simulink model "mySAD_project_full_mission"  (R2023b)
settings: Solver=ode4  StartTime=0.0  StopTime=tf  FixedStep=t_step  RelTol=1e-3
values from neighbouring files (symbols this model uses):
  A1 = importdata("igrfSg.txt")    [SAD_project_code.m]
  A2 = importdata("igrfSh.txt")    [SAD_project_code.m]
  A_1 = area_face(1)    [SAD_project_code.m]
  A_2 = area_face(2)    [SAD_project_code.m]
  A_3 = area_face(3)    [SAD_project_code.m]
  A_4 = area_face(4)    [SAD_project_code.m]
  A_5 = area_face(5)    [SAD_project_code.m]
  A_6 = area_face(6)    [SAD_project_code.m]
  alpha = [1/6 5/6]    [SAD_project_code.m]
  DCM_eci_per = rotationMatrix(rad2deg(i),rad2deg(OM), rad2deg(om))    [SAD_project_code.m]
  e = 0.0011241    [SAD_project_code.m]
  FS = 50000e-9    (= 5e-05)    [SAD_project_code.m]
  H0 = [g_10 g_11 h_11]'    [SAD_project_code.m]
  h_r_0 = [0,0,0]'    [SAD_project_code.m]
  horizon_cone_limit = deg2rad(350)    [SAD_project_code.m]
  I = 5/12.*diag([Ix Iy Iz])    [SAD_project_code.m]
  i = deg2rad(97.55)    [SAD_project_code.m]
  I_inv = inv(I)    [SAD_project_code.m]
  I_RW = 1e-2    (= 0.01)    [SAD_project_code.m]
  I_vector_RW = [I_RW I_RW I_RW]'    [SAD_project_code.m]
  inc_tot = sqrt(inc_lin^2 + inc_acc^2)    [SAD_project_code.m]
  InitialTrueAnomalyOfEarth = 0    [SAD_project_code.m]
  j_b = [0.001 0.005 0.001]'    [SAD_project_code.m]
  K1_point = lqr(A, B, Q, R)    [SAD_project_code.m]
  K1_slew = lqr(A,B, Q, R)    [SAD_project_code.m]
  K2_point = K1_point.^2/2    [SAD_project_code.m]
  K2_slew = K1_slew.^2/2    [SAD_project_code.m]
  K_detumbling = lqr(A,B,Q,R)    [SAD_project_code.m]
  matrix_RW_config = eye(3)    [SAD_project_code.m]
  matrix_RW_config_inv = inv(matrix_RW_config)    [SAD_project_code.m]
  mu_E = astroConstants(13)    [SAD_project_code.m]
  N_1 = BODY(1,:)    [SAD_project_code.m]
  N_2 = BODY(2,:)    [SAD_project_code.m]
  N_3 = BODY(3,:)    [SAD_project_code.m]
  N_4 = BODY(4,:)    [SAD_project_code.m]
  N_5 = BODY(5,:)    [SAD_project_code.m]
  N_6 = BODY(6,:)    [SAD_project_code.m]
  n_e = sqrt(mu_E/a^3)    [SAD_project_code.m]
  N_order = 4    [SAD_project_code.m]
  om = deg2rad(206.3209)    [SAD_project_code.m]
  OM = deg2rad(50.7464)    [SAD_project_code.m]
  p = a*(1-e^2)    [SAD_project_code.m]
  q0 = [0.1, -0.7, 0.51, 0.41]    [SAD_project_code.m]
  r_1 = r(1,:)    [SAD_project_code.m]
  r_2 = r(2,:)    [SAD_project_code.m]
  r_3 = r(3,:)    [SAD_project_code.m]
  r_4 = r(4,:)    [SAD_project_code.m]
  r_5 = r(5,:)    [SAD_project_code.m]
  r_6 = r(6,:)    [SAD_project_code.m]
  R_E = astroConstants(23)    [SAD_project_code.m]
  rho_d1 = 0.1    [SAD_project_code.m]
  rho_d2 = 0.1    [SAD_project_code.m]
  rho_d3 = 0.1    [SAD_project_code.m]
  rho_d4 = 0.1    [SAD_project_code.m]
  rho_d5 = 0.1    [SAD_project_code.m]
  rho_d6 = 0.1    [SAD_project_code.m]
  rho_s1 = rho_s(1)    [SAD_project_code.m]
  rho_s2 = rho_s(2)    [SAD_project_code.m]
  rho_s3 = rho_s(3)    [SAD_project_code.m]
  rho_s4 = rho_s(4)    [SAD_project_code.m]
  rho_s5 = rho_s(5)    [SAD_project_code.m]
  rho_s6 = rho_s(6)    [SAD_project_code.m]
  t_step = 0.01    [SAD_project_code.m]
  th0 = deg2rad(0)    [SAD_project_code.m]
  timeoflaunch = date2mjd2000(date0)    [SAD_project_code.m]
  torque_max = 0.8    [SAD_project_code.m]
  ts_sensor = 5*t_step    (= 0.05)    [SAD_project_code.m]
  w0 = [wx0 wy0 wz0]'    [SAD_project_code.m]
  w0_RW = [0 0 0]    [SAD_project_code.m]
  w_E = deg2rad(15.04)/60/60    [SAD_project_code.m]
  wMax_RW = 2*pi * RPM_max_RW / 60    (= 527.263967027)    [SAD_project_code.m]
libraries: matrix_library x31, simulink_extras x6, sharedtransform x5, simulink x3, dspindex x3, vrlib x2, dspinverses x1, aerolibutil x1
(part 2 of 4)

== system mySAD_project_full_mission/Reaction Wheel Actuator/detect if the RW is saturated (output == 1 isSaturated) ==
  w : Inport
  Abs : Abs  SaturateOnIntegerOverflow=off
  Compare To Constant : simulink/Logic and Bit Operations/Compare To Constant  relop=>=  const=wMax_RW  OutDataTypeStr=boolean
  Demux : Demux  Outputs=3
  Logical Operator : Logic  Operator=OR  AllPortsSameDT=off  OutDataTypeStr=boolean
  Logical Operator1 : Logic  Operator=OR  AllPortsSameDT=off  OutDataTypeStr=boolean
  Logical Operator2 : Logic  Operator=OR  AllPortsSameDT=off  OutDataTypeStr=boolean
  Unit Delay : UnitDelay  SampleTime=-1  HasFrameUpgradeWarning=on
  Unit Delay2 : UnitDelay  SampleTime=-1  HasFrameUpgradeWarning=on
  Unit Delay4 : UnitDelay  SampleTime=-1  HasFrameUpgradeWarning=on
  flag RW1 : Outport
  flag RW2 : Outport  Port=2
  flag RW3 : Outport  Port=3
  wires:
  Unit Delay4/1 -> Logical Operator2/2
  Unit Delay/1 -> Logical Operator/2
  Demux/1 -> Logical Operator/1
  Logical Operator/1 -> flag RW1/1, Unit Delay/1
  Unit Delay2/1 -> Logical Operator1/2
  Logical Operator2/1 -> flag RW3/1, Unit Delay4/1
  Demux/2 -> Logical Operator1/1
  Logical Operator1/1 -> flag RW2/1, Unit Delay2/1
  Demux/3 -> Logical Operator2/1
  Abs/1 -> Compare To Constant/1
  w/1 -> Abs/1
  Compare To Constant/1 -> Demux/1

== system mySAD_project_full_mission/Attitude determination and sensoring/Horizon Sensor1/Normalize Vector1 ==
  Vector : Inport
  Divide : Product  Inputs=*/
  Normalize Vector : Subsystem  AncestorBlock=LibrarySAD5/Normalize Vector1
  Versor : Outport
  wires:
  Vector/1 -> Normalize Vector/1(Vector), Divide/1
  Divide/1 -> Versor/1
  Normalize Vector/1(Norm) -> Divide/2

== system mySAD_project_full_mission/Attitude determination and sensoring/Horizon Sensor1/Normalize Vector2 ==
  Vector : Inport
  Divide : Product  Inputs=*/
  Normalize Vector : Subsystem  AncestorBlock=LibrarySAD5/Normalize Vector1
  Versor : Outport
  wires:
  Vector/1 -> Normalize Vector/1(Vector), Divide/1
  Divide/1 -> Versor/1
  Normalize Vector/1(Norm) -> Divide/2

== system mySAD_project_full_mission/Attitude determination and sensoring/Horizon Sensor1/True Roll and Pitch betwen nadir and -z_body ==
  note: credo inutili e sbagliati
  R_b : Inport
  cone_limit_angle : Inport  Port=2
  Abs2 : Abs  SaturateOnIntegerOverflow=off
  Asin : Trigonometry  Operator=asin
  Asin1 : Trigonometry  Operator=asin
  Asin2 : Trigonometry  Operator=acos
  By defintion : Gain  Gain=-1
  Display : Display
  Display1 : Display
  Display2 : Display
  Dot Product : DotProduct  OutDataTypeStr=Inherit: Inherit via internal rule
  Dot Product1 : DotProduct  OutDataTypeStr=Inherit: Inherit via internal rule
  Dot Product2 : DotProduct  OutDataTypeStr=Inherit: Inherit via internal rule
  Equal2 : RelationalOperator  Operator=<  OutDataTypeStr=boolean  RndMeth=Simplest  InputSameDT=off
  Normalize Vector1 : Subsystem
  Radians to Degrees : simulink_extras/Transformations/Radians to Degrees
  Radians to Degrees1 : simulink_extras/Transformations/Radians to Degrees
  Radians to Degrees2 : simulink_extras/Transformations/Radians to Degrees
  x_b in body frame : Constant  Value=[1,0,0]'
  y_b in body frame1 : Constant  Value=[0,1,0]'
  z_b : Constant  Value=[0 0 1]
  Pitch : Outport
  Roll : Outport  Port=2
  Flag SensorSeeEarth : Outport  Port=3
  wires:
  Dot Product1/1 -> Asin1/1
  R_b/1 -> Normalize Vector1/1(Vector)
  x_b in body frame/1 -> Dot Product/1
  y_b in body frame1/1 -> Dot Product1/1
  Dot Product/1 -> Asin/1
  By defintion/1 -> Radians to Degrees/1
  Asin/1 -> By defintion/1
  Asin1/1 -> Radians to Degrees1/1
  Radians to Degrees1/1 -> Roll/1
  Radians to Degrees/1 -> Pitch/1
  Normalize Vector1/1(Versor) -> Dot Product2/1, Dot Product1/2, Dot Product/2
  z_b/1 -> Dot Product2/2
  Dot Product2/1 -> Asin2/1
  cone_limit_angle/1 -> Display1/1, Equal2/2  "cone max angle"
  Asin2/1 -> Abs2/1
  Abs2/1 -> Radians to Degrees2/1, Equal2/1
  Equal2/1 -> Display2/1, Flag SensorSeeEarth/1
  Radians to Degrees2/1 -> Display/1

== system mySAD_project_full_mission/Attitude determination and sensoring/Subsystem1/If Action Subsystem ==
  Attitude method choice : Inport
  Flag horizon : Inport  Port=2
  Action Port : ActionPort  PropagateVarSize=During execution  ActionPortLabel=else
  Constant : Constant
  Switch : Switch  Criteria=u2 > Threshold  SaturateOnIntegerOverflow=off  InputSameDT=off
  Output : Outport
  wires:
  Attitude method choice/1 -> Switch/1
  Flag horizon/1 -> Switch/2
  Constant/1 -> Switch/3
  Switch/1 -> Output/1

== system mySAD_project_full_mission/Attitude determination and sensoring/Subsystem1/If Action Subsystem1 ==
  Action Port : ActionPort  PropagateVarSize=During execution  ActionPortLabel="if(u1  == 1)"
  Constant : Constant
  Out1 : Outport
  wires:
  Constant/1 -> Out1/1

== system mySAD_project_full_mission/Attitude determination and sensoring/Subsystem1/Switch Case Action Only-Magnetometer ==
  B_b sensor : Inport
  B_N : Inport  Port=2
  w_true : Inport  Port=3
  Action Port : ActionPort  ActionPortLabel=case [ 1 ]:
  Subsystem : Subsystem
  q (scalar last) : Outport
  wires:
  Subsystem/1(q (scalar last)) -> q (scalar last)/1
  B_b sensor/1 -> Subsystem/1(B_b sensor)
  B_N/1 -> Subsystem/2(B_N)
  w_true/1 -> Subsystem/3(Omega True)

== system mySAD_project_full_mission/Attitude determination and sensoring/Subsystem1/Switch Case Action Statisitcal Attitude ==
  B_b sensor : Inport
  Horizon_b sensor : Inport  Port=2
  B_N : Inport  Port=3
  Horizon_N : Inport  Port=4
  Action Port : ActionPort  ActionPortLabel=case [ 2 ]:
  Constant1 : Constant  Value=alpha
  Create matrix to statistical method : Subsystem
  "Statistical methods attitude determination (quaternion  Wabha’s problem) " : Subsystem
  Out1 : Outport
  wires:
  "Statistical methods attitude determination (quaternion  Wabha’s problem) "/1(q in quaternion (scalar last)) -> Out1/1
  Create matrix to statistical method/2(V matrix (inertia)) -> "Statistical methods attitude determination (quaternion  Wabha’s problem) "/3(v matrix)  "V matrix"
  Constant1/1 -> "Statistical methods attitude determination (quaternion  Wabha’s problem) "/1(alpha (weigh of sensor))  "alpha"
  Create matrix to statistical method/1(S matrix (body)) -> "Statistical methods attitude determination (quaternion  Wabha’s problem) "/2(s matrix)  "S matrix"
  B_N/1 -> Create matrix to statistical method/3(Reference1 (Inertial frame))
  B_b sensor/1 -> Create matrix to statistical method/1(Sensor1 (body frame))
  Horizon_N/1 -> Create matrix to statistical method/4(Reference2 (Inertial frame))
  Horizon_b sensor/1 -> Create matrix to statistical method/2(Sensor2 (body frame))

== system mySAD_project_full_mission/Attitude determination and sensoring/Subsystem1/Switch Case Action Triad Case ==
  B_b sensor : Inport
  Horizon_b sensor : Inport  Port=2
  B_N : Inport  Port=3
  Horizon_N : Inport  Port=4
  Action Port : ActionPort  PropagateVarSize=During execution  ActionPortLabel=default:
  DCM to quaternion1 : Subsystem
  TRIAD: Attitude determination algebric Method with 2 sensor : Subsystem
  Output : Outport
  wires:
  B_b sensor/1 -> TRIAD: Attitude determination algebric Method with 2 sensor/1(Sensor1 (body frame))
  Horizon_b sensor/1 -> TRIAD: Attitude determination algebric Method with 2 sensor/2(Sensor2 (body frame))
  B_N/1 -> TRIAD: Attitude determination algebric Method with 2 sensor/3(Reference1 (Inertial frame))
  Horizon_N/1 -> TRIAD: Attitude determination algebric Method with 2 sensor/4(Reference2 (Inertial frame))
  TRIAD: Attitude determination algebric Method with 2 sensor/1(DCM_B/N  Att Det) -> DCM to quaternion1/1(DCM)
  DCM to quaternion1/1(q (scalar last)1) -> Output/1

== system mySAD_project_full_mission/Attitude determination and sensoring/Subsystem1/time derivative ==
  q : Inport
  Gain1 : Gain  Gain=1/ ts_sensor
  Subtract : Sum  Inputs=+-
  Unit Delay : UnitDelay  InitialCondition=[0 0 0 1]'  SampleTime=-1  HasFrameUpgradeWarning=on
  q_dot Versor : Outport
  wires:
  q/1 -> Subtract/1, Unit Delay/1
  Unit Delay/1 -> Subtract/2
  Subtract/1 -> Gain1/1  "dot"
  Gain1/1 -> q_dot Versor/1

== system mySAD_project_full_mission/Calculation of disturbance torque/M of gravity gradient1/Norm of vector ==
  Vector : Inport
  Dot Product : DotProduct  OutDataTypeStr=Inherit: Inherit via internal rule
  Sqrt : Sqrt
  Norm : Outport
  wires:
  Sqrt/1 -> Norm/1
  Vector/1 -> Dot Product/1, Dot Product/2
  Dot Product/1 -> Sqrt/1

== system mySAD_project_full_mission/Calculation of disturbance torque/Solar pressure on 6 faces/Norm of vector ==
  Vector : Inport
  Dot Product : DotProduct  OutDataTypeStr=Inherit: Inherit via internal rule
  Sqrt : Sqrt
  Norm : Outport
  wires:
  Sqrt/1 -> Norm/1
  Vector/1 -> Dot Product/1, Dot Product/2
  Dot Product/1 -> Sqrt/1

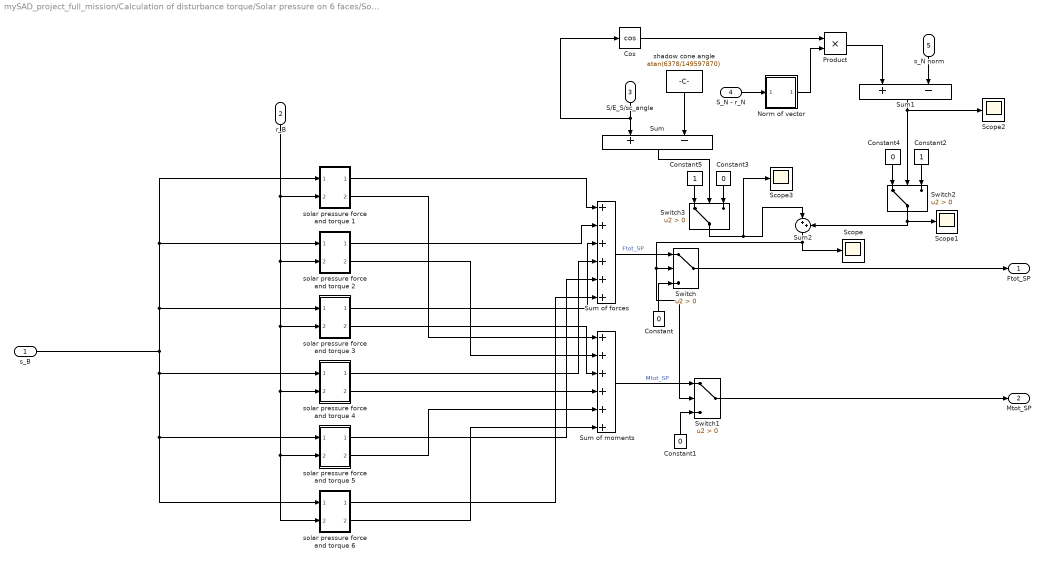
== system mySAD_project_full_mission/Calculation of disturbance torque/Solar pressure on 6 faces/Solar pressure on 6 faces1 ==
  s_B : Inport
  r_B : Inport  Port=2
  S/E_S/sc_angle : Inport  Port=3
  S_N - r_N : Inport  Port=4
  s_N norm : Inport  Port=5
  Constant{,1,3..4} (4 alike) : Constant  Value=0
  Constant2 : Constant
  Constant5 : Constant
  Cos : Trigonometry  Operator=cos
  Norm of vector : Subsystem  AncestorBlock=LibrarySAD5/Normalize Vector1
  Product : Product
  Scope{,1..3} (4 alike) : Scope
  Sum : Sum  Inputs=+-
  Sum of forces : Sum  Inputs=++++++
  Sum of moments : Sum  Inputs=++++++
  Sum1 : Sum  Inputs=+-
  Sum2 : Sum  Inputs=|++
  Switch{,1..3} (4 alike) : Switch  Criteria=u2 > Threshold  SaturateOnIntegerOverflow=off  InputSameDT=off
  shadow cone angle : Constant  Value=atan(6378/149597870)
  solar pressure force and torque 1 : Subsystem
  solar pressure force and torque 2 : Subsystem
  solar pressure force and torque 3 : Subsystem
  solar pressure force and torque 4 : Subsystem
  solar pressure force and torque 5 : Subsystem
  solar pressure force and torque 6 : Subsystem
  Ftot_SP : Outport
  Mtot_SP : Outport  Port=2
  wires:
  s_B/1 -> solar pressure force and torque 1/1(s_B), solar pressure force and torque 2/1(s_B), solar pressure force and torque 3/1(s_B), solar pressure force and torque 4/1(s_B), solar pressure force and torque 6/1(s_B), solar pressure force and torque 5/1(s_B)
  solar pressure force and torque 1/1(F_1) -> Sum of forces/1
  solar pressure force and torque 1/2(M_1) -> Sum of moments/1
  solar pressure force and torque 2/1(F_2) -> Sum of forces/2
  r_B/1 -> solar pressure force and torque 6/2(r_N), solar pressure force and torque 5/2(r_N), solar pressure force and torque 4/2(r_N), solar pressure force and torque 3/2(r_N), solar pressure force and torque 2/2(r_N), solar pressure force and torque 1/2(r_N)
  solar pressure force and torque 2/2(M_2) -> Sum of moments/2
  solar pressure force and torque 3/1(F_3) -> Sum of forces/3
  solar pressure force and torque 3/2(M_3) -> Sum of moments/3
  solar pressure force and torque 4/1(F_4) -> Sum of forces/4
  solar pressure force and torque 4/2(M_4) -> Sum of moments/4
  solar pressure force and torque 5/1(F_5) -> Sum of forces/5
  solar pressure force and torque 5/2(M_5) -> Sum of moments/5
  solar pressure force and torque 6/1(F_6) -> Sum of forces/6
  solar pressure force and torque 6/2(M_6) -> Sum of moments/6
  Sum of forces/1 -> Switch/1  "Ftot_SP"
  Constant/1 -> Switch/3
  S/E_S/sc_angle/1 -> Cos/1, Sum/1
  shadow cone angle/1 -> Sum/2
  Sum of moments/1 -> Switch1/1  "Mtot_SP"
  Constant1/1 -> Switch1/3
  S_N - r_N/1 -> Norm of vector/1(Vector)
  Constant2/1 -> Switch2/3
  Cos/1 -> Product/1
  Norm of vector/1(Norm) -> Product/2
  Product/1 -> Sum1/1
  s_N norm/1 -> Sum1/2
  Sum/1 -> Switch3/2
  Sum1/1 -> Switch2/2, Scope2/1
  Constant4/1 -> Switch2/1
  Constant5/1 -> Switch3/1
  Constant3/1 -> Switch3/3
  Switch3/1 -> Scope3/1, Sum2/1
  Switch2/1 -> Sum2/2, Scope1/1
  Sum2/1 -> Scope/1, Switch1/2, Switch/2
  Switch/1 -> Ftot_SP/1
  Switch1/1 -> Mtot_SP/1

== system mySAD_project_full_mission/Determine Control algorithm/Switch Case Action 3 axis stabilization Algorithm/Check if the Mc is finite ==
  Mc : Inport
  Constant : Constant  Value=[0,0,0]'
  IsNaN : RelationalOperator  Operator=isNaN  OutDataTypeStr=boolean  RndMeth=Simplest  InputSameDT=off
  Norm vector : Subsystem  AncestorBlock=LibrarySAD5/Normalize Vector1
  Switch : Switch  Criteria=u2 > Threshold  SaturateOnIntegerOverflow=off  InputSameDT=off
  Control Moment : Outport
  wires:
  Constant/1 -> Switch/1
  IsNaN/1 -> Norm vector/1(Vector)
  Norm vector/1(Norm) -> Switch/2
  Mc/1 -> Switch/3, IsNaN/1
  Switch/1 -> Control Moment/1

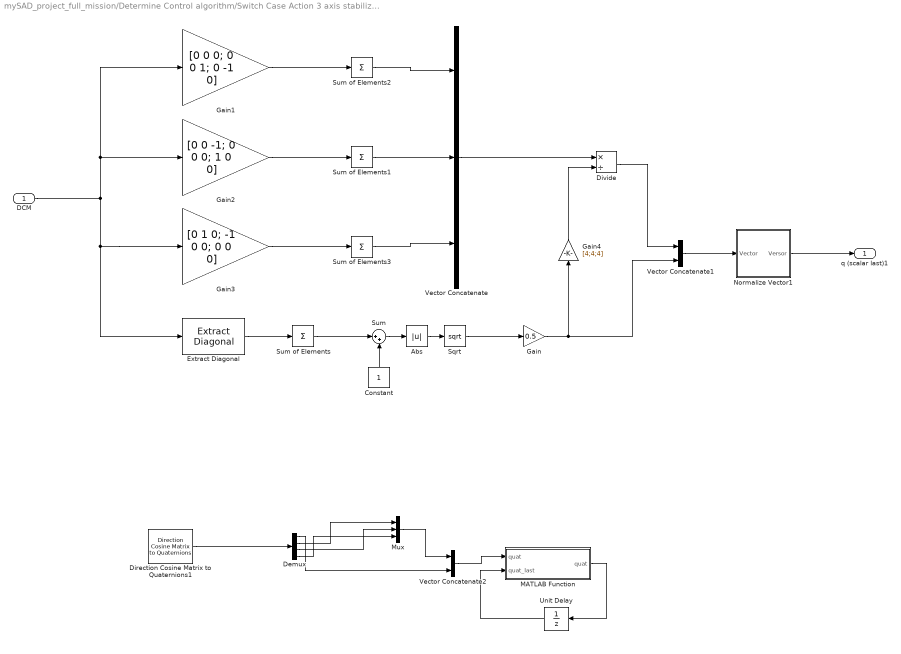
== system mySAD_project_full_mission/Determine Control algorithm/Switch Case Action 3 axis stabilization Algorithm/DCM to quaternion1 ==
  DCM : Inport
  Abs : Abs  SaturateOnIntegerOverflow=off
  Constant : Constant
  Demux : Demux
  Direction Cosine Matrix to Quaternions1 : sharedtransform/Direction Cosine Matrix  to Quaternions  aMode=0  action=None  tolerance=eps(2)
      settings: LibrarySourceBlock=|
      | aerolibtransform2/Direction Cosine Matrix
      | to Quaternions
  Divide : Product  Inputs=*/
  Extract Diagonal : matrix_library/Extract Diagonal
      settings: LibrarySourceBlock=|
      | simulink/Matrix
      | Operations/Extract Diagonal
  Gain : Gain  Gain=0.5
  Gain1 : Gain  Gain=[0 0 0; 0 0 1; 0 -1 0]
  Gain2 : Gain  Gain=[0 0 -1; 0 0 0; 1 0 0]
  Gain3 : Gain  Gain=[0 1 0; -1 0 0; 0 0 0]
  Gain4 : Gain  Gain=[4;4;4]
  MATLAB Function : MATLAB Function  TreatAsAtomicUnit=on
  Mux : Mux  Inputs=3
  Normalize Vector1 : Subsystem
  Sqrt : Sqrt
  Sum : Sum  Inputs=|++
  Sum of Elements{,1..3} (4 alike) : Sum  Inputs=+
  Unit Delay : UnitDelay  InitialCondition=q0  SampleTime=-1  HasFrameUpgradeWarning=on
  Vector Concatenate : Concatenate  NumInputs=3
  Vector Concatenate1 : Concatenate
  Vector Concatenate2 : Concatenate
  q (scalar last)1 : Outport
  wires:
  Extract Diagonal/1 -> Sum of Elements/1
  Sum of Elements/1 -> Sum/1
  Constant/1 -> Sum/2
  Sqrt/1 -> Gain/1
  DCM/1 -> Gain1/1, Gain2/1, Gain3/1, Extract Diagonal/1
  Gain2/1 -> Sum of Elements1/1
  Sum of Elements1/1 -> Vector Concatenate/2
  Gain1/1 -> Sum of Elements2/1
  Sum of Elements2/1 -> Vector Concatenate/1
  Sum of Elements3/1 -> Vector Concatenate/3
  Gain3/1 -> Sum of Elements3/1
  Vector Concatenate/1 -> Divide/1
  Gain/1 -> Vector Concatenate1/2, Gain4/1
  Divide/1 -> Vector Concatenate1/1
  Vector Concatenate1/1 -> Normalize Vector1/1(Vector)
  Sum/1 -> Abs/1
  Gain4/1 -> Divide/2
  Abs/1 -> Sqrt/1
  Direction Cosine Matrix to Quaternions1/1 -> Demux/1
  Demux/2 -> Mux/1
  Demux/3 -> Mux/2
  Demux/4 -> Mux/3
  Demux/1 -> Vector Concatenate2/2
  Mux/1 -> Vector Concatenate2/1
  Vector Concatenate2/1 -> MATLAB Function/1("quat ")
  Unit Delay/1 -> MATLAB Function/2(quat_last)
  MATLAB Function/1(quat) -> Unit Delay/1
  Normalize Vector1/1(Versor) -> q (scalar last)1/1

== system mySAD_project_full_mission/Determine Control algorithm/Switch Case Action 3 axis stabilization Algorithm/Relative attitude error quaternion3 ==
  q1 (usually Target) : Inport
  q2 (Estimated) : Inport  Port=2
  Demux : Demux
  Gain1 : Gain  Gain=[0,0,0,-1; 0,0,1,0; 0,-1,0 0; 1,0,0,0]
  Gain2 : Gain  Gain=[0, 0, -1 ,0; 0, 0 ,0 ,-1; 1, 0, 0, 0; 0 1, 0, 0]
  Gain3 : Gain  Gain=[0 1 0 0; -1 0 0 0; 0 0 0 -1; 0 0 1 0]
  Gain4 : Gain  Gain=eye(4)
  Matrix Multiply : Product  Multiplication=Matrix(*)
  Sum1 : Sum  Inputs=++++
  qe : Outport
  wires:
  Gain1/1 -> Sum1/1
  Demux/2 -> Gain2/1
  Gain3/1 -> Sum1/3
  Demux/1 -> Gain1/1
  Sum1/1 -> Matrix Multiply/1
  Demux/3 -> Gain3/1
  Gain4/1 -> Sum1/4
  Gain2/1 -> Sum1/2
  Demux/4 -> Gain4/1
  q2 (Estimated)/1 -> Matrix Multiply/2
  Matrix Multiply/1 -> qe/1
  q1 (usually Target)/1 -> Demux/1

== system mySAD_project_full_mission/Determine Control algorithm/Switch Case Action Slew Maneuver Algorithm/Check if the Mc is finite ==
  Mc : Inport
  Constant : Constant  Value=[0,0,0]'
  IsNaN : RelationalOperator  Operator=isNaN  OutDataTypeStr=boolean  RndMeth=Simplest  InputSameDT=off
  Norm vector : Subsystem  AncestorBlock=LibrarySAD5/Normalize Vector1
  Switch : Switch  Criteria=u2 > Threshold  SaturateOnIntegerOverflow=off  InputSameDT=off
  Control Moment : Outport
  wires:
  Constant/1 -> Switch/1
  IsNaN/1 -> Norm vector/1(Vector)
  Norm vector/1(Norm) -> Switch/2
  Mc/1 -> Switch/3, IsNaN/1
  Switch/1 -> Control Moment/1

== system mySAD_project_full_mission/Determine Control algorithm/Switch Case Action Slew Maneuver Algorithm/DCM to quaternion1 ==
  DCM : Inport
  Abs : Abs  SaturateOnIntegerOverflow=off
  Constant : Constant
  Demux : Demux
  Direction Cosine Matrix to Quaternions1 : sharedtransform/Direction Cosine Matrix  to Quaternions  aMode=0  action=None  tolerance=eps(2)
      settings: LibrarySourceBlock=|
      | aerolibtransform2/Direction Cosine Matrix
      | to Quaternions
  Divide : Product  Inputs=*/
  Extract Diagonal : matrix_library/Extract Diagonal
      settings: LibrarySourceBlock=|
      | simulink/Matrix
      | Operations/Extract Diagonal
  Gain : Gain  Gain=0.5
  Gain1 : Gain  Gain=[0 0 0; 0 0 1; 0 -1 0]
  Gain2 : Gain  Gain=[0 0 -1; 0 0 0; 1 0 0]
  Gain3 : Gain  Gain=[0 1 0; -1 0 0; 0 0 0]
  Gain4 : Gain  Gain=[4;4;4]
  Guarantee sign continuity for quaternion : MATLAB Function  TreatAsAtomicUnit=on
  Mux : Mux  Inputs=3
  Normalize Vector1 : Subsystem
  Sqrt : Sqrt
  Sum : Sum  Inputs=|++
  Sum of Elements{,1..3} (4 alike) : Sum  Inputs=+
  Unit Delay : UnitDelay  InitialCondition=[0,0,0,1]  SampleTime=-1  HasFrameUpgradeWarning=on
  Vector Concatenate : Concatenate  NumInputs=3
  Vector Concatenate1 : Concatenate
  Vector Concatenate2 : Concatenate
  q (scalar last)1 : Outport
  wires:
  Extract Diagonal/1 -> Sum of Elements/1
  Sum of Elements/1 -> Sum/1
  Constant/1 -> Sum/2
  Sqrt/1 -> Gain/1
  DCM/1 -> Gain1/1, Gain2/1, Gain3/1, Extract Diagonal/1
  Gain2/1 -> Sum of Elements1/1
  Sum of Elements1/1 -> Vector Concatenate/2
  Gain1/1 -> Sum of Elements2/1
  Sum of Elements2/1 -> Vector Concatenate/1
  Sum of Elements3/1 -> Vector Concatenate/3
  Gain3/1 -> Sum of Elements3/1
  Vector Concatenate/1 -> Divide/1
  Gain/1 -> Vector Concatenate1/2, Gain4/1
  Divide/1 -> Vector Concatenate1/1
  Vector Concatenate1/1 -> Normalize Vector1/1(Vector)
  Sum/1 -> Abs/1
  Gain4/1 -> Divide/2
  Abs/1 -> Sqrt/1
  Direction Cosine Matrix to Quaternions1/1 -> Demux/1
  Demux/2 -> Mux/1
  Demux/3 -> Mux/2
  Demux/4 -> Mux/3
  Demux/1 -> Vector Concatenate2/2
  Mux/1 -> Vector Concatenate2/1
  Vector Concatenate2/1 -> Guarantee sign continuity for quaternion/1("quat ")
  Unit Delay/1 -> Guarantee sign continuity for quaternion/2(quat_last)
  Guarantee sign continuity for quaternion/1(quat) -> Unit Delay/1
  Normalize Vector1/1(Versor) -> q (scalar last)1/1

== system mySAD_project_full_mission/Determine Control algorithm/Switch Case Action Slew Maneuver Algorithm/Relative attitude error quaternion3 ==
  q1 (usually Target) : Inport
  q2 (Estimated) : Inport  Port=2
  Demux : Demux
  Gain1 : Gain  Gain=[0,0,0,-1; 0,0,1,0; 0,-1,0 0; 1,0,0,0]
  Gain2 : Gain  Gain=[0, 0, -1 ,0; 0, 0 ,0 ,-1; 1, 0, 0, 0; 0 1, 0, 0]
  Gain3 : Gain  Gain=[0 1 0 0; -1 0 0 0; 0 0 0 -1; 0 0 1 0]
  Gain4 : Gain  Gain=eye(4)
  Matrix Multiply : Product  Multiplication=Matrix(*)
  Sum1 : Sum  Inputs=++++
  qe : Outport
  wires:
  Gain1/1 -> Sum1/1
  Demux/2 -> Gain2/1
  Gain3/1 -> Sum1/3
  Demux/1 -> Gain1/1
  Sum1/1 -> Matrix Multiply/1
  Demux/3 -> Gain3/1
  Gain4/1 -> Sum1/4
  Gain2/1 -> Sum1/2
  Demux/4 -> Gain4/1
  q2 (Estimated)/1 -> Matrix Multiply/2
  Matrix Multiply/1 -> qe/1
  q1 (usually Target)/1 -> Demux/1

== system mySAD_project_full_mission/Determine Control algorithm/Switch Case Action Slew Maneuver Algorithm/cross(w, Iw) ==
  w : Inport
  Inertia : Inport  Port=2
  Cross Product : matrix_library/Cross Product
  Matrix Multiply : Product  Multiplication=Matrix(*)
  "cross(w, Iw)" : Outport
  wires:
  Cross Product/1 -> "cross(w, Iw)"/1
  w/1 -> Matrix Multiply/2, Cross Product/1
  Matrix Multiply/1 -> Cross Product/2
  Inertia/1 -> Matrix Multiply/1

== system mySAD_project_full_mission/Dynamics e Kinematics/Attitude error GG/calculating A_B//L ==
  Theta : Inport
  A_B/N : Inport  Port=2
  Matrix Multiply : Product  Multiplication=Matrix(*)
  Subsystem : Subsystem
  Transpose : Math  Operator=transpose
  A_B/L : Outport
  A_L/N : Outport  Port=2
  wires:
  Theta/1 -> Subsystem/1(Theta)
  Transpose/1 -> Matrix Multiply/2
  A_B/N/1 -> Matrix Multiply/1
  Matrix Multiply/1 -> A_B/L/1
  Subsystem/1(" A_L/N") -> A_L/N/1, Transpose/1

== system mySAD_project_full_mission/Dynamics e Kinematics/DCM composition from quaternions 1/Cross product matrix composition ==
  q_vect : Inport
  Demux : Demux  Outputs=3
  Gain : Gain  Gain=[0 0 0; 0 0 -1; 0 1 0]
  Gain1 : Gain  Gain=[0 0 1; 0 0 0; -1 0 0]
  Gain2 : Gain  Gain=[0 -1 0; 1 0 0; 0 0 0]
  Sum : Sum  Inputs=+++
  q_vect cross : Outport
  wires:
  Gain1/1 -> Sum/2
  Demux/3 -> Gain2/1
  Demux/1 -> Gain/1
  q_vect/1 -> Demux/1
  Gain2/1 -> Sum/3
  Demux/2 -> Gain1/1
  Gain/1 -> Sum/1
  Sum/1 -> q_vect cross/1

== system mySAD_project_full_mission/Dynamics e Kinematics/Kinematics quaternion2/Matrix OMEGA ==
  omega : Inport
  Constant4 : Constant  Value=0
  Demux : Demux  Outputs=3
  Gain : Gain  Gain=-1
  Gain1 : Gain  Gain=-1
  Gain2 : Gain  Gain=-1
  Matrix Concatenate : Concatenate  NumInputs=4  Mode=Multidimensional array  ConcatenateDimension=2
  Vector Concatenate{,2..4} (4 alike) : Concatenate  NumInputs=4
  Matrix Omega : Outport
  wires:
  Demux/2 -> Vector Concatenate4/2, Vector Concatenate/3, Gain1/1  "W_v"
  Gain1/1 -> Vector Concatenate2/4, Vector Concatenate3/1
  Matrix Concatenate/1 -> Matrix Omega/1
  Gain2/1 -> Vector Concatenate3/4, Vector Concatenate/2  "-W_w"
  Vector Concatenate3/1 -> Matrix Concatenate/3
  Demux/3 -> Vector Concatenate2/1, Vector Concatenate4/3, Gain2/1  "W_w"
  Gain/1 -> Vector Concatenate/4, Vector Concatenate2/3  "-W_u"
  Constant4/1 -> Vector Concatenate/1, Vector Concatenate2/2, Vector Concatenate3/3, Vector Concatenate4/4
  Demux/1 -> Vector Concatenate3/2, Vector Concatenate4/1, Gain/1  "W_u"
  Vector Concatenate4/1 -> Matrix Concatenate/4
  Vector Concatenate2/1 -> Matrix Concatenate/2
  Vector Concatenate/1 -> Matrix Concatenate/1
  omega/1 -> Demux/1

== system mySAD_project_full_mission/Dynamics e Kinematics/Kinematics quaternion2/Normalize Vector2 ==
  Vector : Inport
  Dot Product : DotProduct  OutDataTypeStr=Inherit: Inherit via internal rule
  Sqrt : Sqrt
  Norm : Outport
  wires:
  Sqrt/1 -> Norm/1
  Vector/1 -> Dot Product/1, Dot Product/2
  Dot Product/1 -> Sqrt/1

== system mySAD_project_full_mission/Enviroment Model/Magnetic Field/Switch Case Action Adavanced Magnetic model ==
  r_N : Inport
  Action Port : ActionPort  PropagateVarSize=During execution  ActionPortLabel=case [ 1 ]:
  Advanced magnetic field model : Subsystem
  Constant : Constant  Value=N_order
  Gain : Gain  Gain=10^(-9)
  B_n : Outport  VectorParamsAs1DForOutWhenUnconnected=off
  wires:
  r_N/1 -> Advanced magnetic field model/1(r_N)
  Advanced magnetic field model/1(B_n) -> Gain/1
  Gain/1 -> B_n/1
  Constant/1 -> Advanced magnetic field model/2(N order)

== system mySAD_project_full_mission/Enviroment Model/Magnetic Field/Switch Case Action Dipole model ==
  r_N : Inport
  Action Port : ActionPort  PropagateVarSize=During execution  ActionPortLabel=default:
  Dipol Model of Magnetic Field : Subsystem
  Gain : Gain  Gain=10^(-9)
  "[g0_1, g1_1, h1_1]" : Constant  Value=H0
  b_N : Outport  VectorParamsAs1DForOutWhenUnconnected=off
  wires:
  "[g0_1, g1_1, h1_1]"/1 -> Dipol Model of Magnetic Field/1(H0 vector)
  r_N/1 -> Dipol Model of Magnetic Field/2(EarthSat_n)
  Dipol Model of Magnetic Field/1(b_N) -> Gain/1
  Gain/1 -> b_N/1

== system mySAD_project_full_mission/Enviroment Model/two-body Keplerian dynamics ECI/Integretion of true anomaly ==
  th0 : Inport
  (1-e^2)^(3/2) : Subsystem
  Constant : Constant
  Cos : Trigonometry  Operator=cos
  Divide : Product  Inputs=*/
  Gain : Gain  Gain=e
  Gain1 : Gain  Gain=n_e
  Integrator : Integrator  InitialConditionSource=external
  Product : Product
  Sum : Sum  Inputs=|++
  th : Outport
  wires:
  Sum/1 -> Product/1, Product/2
  Integrator/1 -> th/1, Cos/1  "theta"
  Divide/1 -> Integrator/1
  Constant/1 -> Sum/1
  Product/1 -> Gain1/1
  Cos/1 -> Gain/1
  Gain/1 -> Sum/2
  (1-e^2)^(3/2)/1(Out1) -> Divide/2
  th0/1 -> Integrator/2
  Gain1/1 -> Divide/1

== system mySAD_project_full_mission/Enviroment Model/two-body Keplerian dynamics ECI/r_perifocal ==
  th : Inport
  Calculation of norm r : Subsystem
  Constant : Constant  Value=0
  Cos : Trigonometry  Operator=cos
  Mux : Mux  Inputs=3
  Product : Product
  Sin : Trigonometry
  r_per : Outport
  wires:
  Constant/1 -> Mux/3
  Cos/1 -> Mux/1
  th/1 -> Calculation of norm r/1(th), Cos/1, Sin/1
  Sin/1 -> Mux/2
  Mux/1 -> Product/1  "r_n"
  Calculation of norm r/1(Norm(r)) -> Product/2
  Product/1 -> r_per/1  "r_n"

== system mySAD_project_full_mission/Attitude determination and sensoring/Horizon Sensor1/Normalize Vector1/Normalize Vector ==
  Vector : Inport
  Dot Product : DotProduct  OutDataTypeStr=Inherit: Inherit via internal rule
  Sqrt : Sqrt
  Norm : Outport
  wires:
  Sqrt/1 -> Norm/1
  Vector/1 -> Dot Product/1, Dot Product/2
  Dot Product/1 -> Sqrt/1

== system mySAD_project_full_mission/Attitude determination and sensoring/Horizon Sensor1/Normalize Vector2/Normalize Vector ==
  Vector : Inport
  Dot Product : DotProduct  OutDataTypeStr=Inherit: Inherit via internal rule
  Sqrt : Sqrt
  Norm : Outport
  wires:
  Sqrt/1 -> Norm/1
  Vector/1 -> Dot Product/1, Dot Product/2
  Dot Product/1 -> Sqrt/1

== system mySAD_project_full_mission/Attitude determination and sensoring/Horizon Sensor1/True Roll and Pitch betwen nadir and -z_body/Normalize Vector1 ==
  Vector : Inport
  Divide : Product  Inputs=*/
  Normalize Vector : Subsystem  AncestorBlock=LibrarySAD5/Normalize Vector1
  Versor : Outport
  wires:
  Vector/1 -> Normalize Vector/1(Vector), Divide/1
  Divide/1 -> Versor/1
  Normalize Vector/1(Norm) -> Divide/2

== system mySAD_project_full_mission/Attitude determination and sensoring/Subsystem1/Switch Case Action Only-Magnetometer/Subsystem ==
  B_b sensor : Inport
  B_N : Inport  Port=2
  Omega True : Inport  Port=3
  Cross Product4 : matrix_library/Cross Product
  DCM to quaternion1 : Subsystem
  Divide : Product  Inputs=*/
  Gain3 : Gain  Gain=1/ts_sensor
  Matrix Multiply2 : Product  Multiplication=Matrix(*)
  Norm vector : Subsystem  AncestorBlock=LibrarySAD5/Normalize Vector1
  Normalize Vector1 : Subsystem
  Normalize Vector5 : Subsystem
  Scope : Scope
  Square : Math  Operator=square
  Subsystem : Subsystem
  Subsystem1 : Subsystem
  Subtract3 : Sum  Inputs=+-
  Unit Delay : UnitDelay  SampleTime=-1  HasFrameUpgradeWarning=on
  Unit Delay2 : UnitDelay  InitialCondition=[1,0,0]'  SampleTime=-1  HasFrameUpgradeWarning=on
  time derivative : Subsystem
  q (scalar last) : Outport
  wires:
  time derivative/1(B_b dot Versor) -> Norm vector/1(Vector), Unit Delay2/1, Cross Product4/1  "B_b dot"
  Unit Delay2/1 -> Cross Product4/2
  Norm vector/1(Norm) -> Square/1
  Cross Product4/1 -> Divide/1
  Square/1 -> Divide/2
  Divide/1 -> Gain3/1
  Matrix Multiply2/1 -> DCM to quaternion1/1(DCM)
  Normalize Vector1/1(Versor) -> Subsystem/1(B_b versor)  "B_b versor"
  Subsystem/1(b_matrix) -> Matrix Multiply2/1
  Normalize Vector5/1(Versor) -> Subsystem1/1(B_N versor)
  Subsystem1/1(r_matrix) -> Matrix Multiply2/2
  B_N/1 -> Unit Delay/1
  Subtract3/1 -> Scope/1
  Gain3/1 -> Subtract3/2
  Omega True/1 -> Subtract3/1
  B_b sensor/1 -> time derivative/1(B_b), Normalize Vector1/1(Vector)
  DCM to quaternion1/1(q (scalar last)1) -> q (scalar last)/1
  Unit Delay/1 -> Normalize Vector5/1(Vector)

== system mySAD_project_full_mission/Attitude determination and sensoring/Subsystem1/Switch Case Action Statisitcal Attitude/Create matrix to statistical method ==
  Sensor1 (body frame) : Inport
  Sensor2 (body frame) : Inport  Port=2
  Reference1 (Inertial frame) : Inport  Port=3
  Reference2 (Inertial frame) : Inport  Port=4
  Matrix Concatenate1 : Concatenate  Mode=Multidimensional array  ConcatenateDimension=2
  Matrix Concatenate2 : Concatenate  Mode=Multidimensional array  ConcatenateDimension=2
  Normalize Vector1 : Subsystem
  Normalize Vector2 : Subsystem
  Normalize Vector3 : Subsystem
  Normalize Vector4 : Subsystem
  S matrix (body) : Outport
  V matrix (inertia) : Outport  Port=2
  wires:
  Matrix Concatenate1/1 -> V matrix (inertia)/1
  Normalize Vector1/1(Versor) -> Matrix Concatenate2/1
  Normalize Vector2/1(Versor) -> Matrix Concatenate2/2
  Normalize Vector4/1(Versor) -> Matrix Concatenate1/2
  Normalize Vector3/1(Versor) -> Matrix Concatenate1/1
  Matrix Concatenate2/1 -> S matrix (body)/1
  Reference1 (Inertial frame)/1 -> Normalize Vector3/1(Vector)
  Reference2 (Inertial frame)/1 -> Normalize Vector4/1(Vector)
  Sensor1 (body frame)/1 -> Normalize Vector1/1(Vector)
  Sensor2 (body frame)/1 -> Normalize Vector2/1(Vector)

== system mySAD_project_full_mission/Attitude determination and sensoring/Subsystem1/Switch Case Action Statisitcal Attitude/Statistical methods attitude determination (quaternion  Wabha’s problem)  ==
  note: In questo blocco ci sono altri metodi per il calcolo di q
  note: BLOCCO DA SISTEMARE SCEGLIENDO UNA SOLUZIONE
  note: Resolve linear system:
      | (𝑆 − σI)𝑞 + zq_4 = 𝜆_(MAX)*𝑞
      | 𝑧'𝑞 + σ*q_4 = 𝜆_(MAX)*𝑞_4
      |
      | Calculate eigenvalue (in the theory we assumed that lambda_max = 1)
  note: 𝐾 = [ (𝑆 − σI), 𝑧
      | 𝑧 ' 𝜎 ]
  note: 𝑧 = [𝑏23 − 𝑏32 , b31 − 𝑏13 , b12 − 𝑏21] '
  alpha (weigh of sensor) : Inport
  s matrix : Inport  Port=2
  v matrix : Inport  Port=3
  Adjoint of 3x3 Matrix : aerolibutil/Adjoint of 3x3 Matrix
  Blocco da convertire in formato simulink. Ho trovato 3 soluzioni differenti al proble : MATLAB Function  TreatAsAtomicUnit=on
  For Iterator Subsystem to calculate B matrix : Subsystem  TreatAsAtomicUnit=on
  Gain : Gain  Gain=eye(3)
  Matrix Concatenate : Concatenate  Mode=Multidimensional array  ConcatenateDimension=2
  Matrix Concatenate1 : Concatenate  Mode=Multidimensional array
  Matrix trace : Subsystem
  Subtract : Sum  Inputs=+-
  Sum : Sum  Inputs=|++
  Transpose : Math  Operator=transpose
  Transpose2 : Math  Operator=transpose
  Vector Concatenate1 : Concatenate
  Vector z : Subsystem
  q in quaternion (scalar last) : Outport
  wires:
  Transpose/1 -> Sum/2
  For Iterator Subsystem to calculate B matrix/1(B matrix) -> Vector z/1(B), Matrix trace/1(Matrix), Transpose/1, Sum/1  "B matrix"
  Sum/1 -> Adjoint of 3x3 Matrix/1, Blocco da convertire in formato simulink. Ho trovato 3 soluzioni differenti al proble/2(S), Subtract/1  "matrix S"
  Gain/1 -> Subtract/2
  Matrix trace/1(trace) -> Vector Concatenate1/2, Gain/1  "sigma = tr(B)"
  Matrix Concatenate/1 -> Matrix Concatenate1/1
  Vector Concatenate1/1 -> Transpose2/1
  Vector z/1(z) -> Vector Concatenate1/1, Matrix Concatenate/2
  Transpose2/1 -> Matrix Concatenate1/2
  Subtract/1 -> Matrix Concatenate/1  "S - sigma*eye(3)"
  alpha (weigh of sensor)/1 -> For Iterator Subsystem to calculate B matrix/1(alpha)
  v matrix/1 -> For Iterator Subsystem to calculate B matrix/3(v matrix)
  s matrix/1 -> For Iterator Subsystem to calculate B matrix/2(s matrix)
  Blocco da convertire in formato simulink. Ho trovato 3 soluzioni differenti al proble/1(q) -> q in quaternion (scalar last)/1  "q in quaternion (scalar last)"
  Adjoint of 3x3 Matrix/1 -> Blocco da convertire in formato simulink. Ho trovato 3 soluzioni differenti al proble/3(Sadj)
  Matrix Concatenate1/1 -> Blocco da convertire in formato simulink. Ho trovato 3 soluzioni differenti al proble/1(K)  "K matrix"

== system mySAD_project_full_mission/Attitude determination and sensoring/Subsystem1/Switch Case Action Triad Case/DCM to quaternion1 ==
  DCM : Inport
  Abs : Abs  SaturateOnIntegerOverflow=off
  Constant : Constant
  Demux : Demux
  Direction Cosine Matrix to Quaternions1 : sharedtransform/Direction Cosine Matrix  to Quaternions  aMode=0  action=None  tolerance=eps(2)
      settings: LibrarySourceBlock=|
      | aerolibtransform2/Direction Cosine Matrix
      | to Quaternions
  Divide : Product  Inputs=*/
  Extract Diagonal : matrix_library/Extract Diagonal
      settings: LibrarySourceBlock=|
      | simulink/Matrix
      | Operations/Extract Diagonal
  Gain : Gain  Gain=0.5
  Gain1 : Gain  Gain=[0 0 0; 0 0 1; 0 -1 0]
  Gain2 : Gain  Gain=[0 0 -1; 0 0 0; 1 0 0]
  Gain3 : Gain  Gain=[0 1 0; -1 0 0; 0 0 0]
  Gain4 : Gain  Gain=[4;4;4]
  MATLAB Function : MATLAB Function  TreatAsAtomicUnit=on
  Mux : Mux  Inputs=3
  Normalize Vector1 : Subsystem
  Sqrt : Sqrt
  Sum : Sum  Inputs=|++
  Sum of Elements{,1..3} (4 alike) : Sum  Inputs=+
  Unit Delay : UnitDelay  InitialCondition=q0  SampleTime=-1  HasFrameUpgradeWarning=on
  Vector Concatenate : Concatenate  NumInputs=3
  Vector Concatenate1 : Concatenate
  Vector Concatenate2 : Concatenate
  q (scalar last)1 : Outport
  wires:
  Extract Diagonal/1 -> Sum of Elements/1
  Sum of Elements/1 -> Sum/1
  Constant/1 -> Sum/2
  Sqrt/1 -> Gain/1
  ? -> Gain1/1, Gain2/1, Gain3/1, Extract Diagonal/1
  Gain2/1 -> Sum of Elements1/1
  Sum of Elements1/1 -> Vector Concatenate/2
  Gain1/1 -> Sum of Elements2/1
  Sum of Elements2/1 -> Vector Concatenate/1
  Sum of Elements3/1 -> Vector Concatenate/3
  Gain3/1 -> Sum of Elements3/1
  Vector Concatenate/1 -> Divide/1
  Gain/1 -> Vector Concatenate1/2, Gain4/1
  Divide/1 -> Vector Concatenate1/1
  Vector Concatenate1/1 -> Normalize Vector1/1(Vector)
  Sum/1 -> Abs/1
  Gain4/1 -> Divide/2
  Abs/1 -> Sqrt/1
  Direction Cosine Matrix to Quaternions1/1 -> Demux/1
  Demux/2 -> Mux/1
  Demux/3 -> Mux/2
  Demux/4 -> Mux/3
  Demux/1 -> Vector Concatenate2/2
  Mux/1 -> Vector Concatenate2/1
  DCM/1 -> Direction Cosine Matrix to Quaternions1/1
  Vector Concatenate2/1 -> MATLAB Function/1("quat ")
  Unit Delay/1 -> MATLAB Function/2(quat_last)
  MATLAB Function/1(quat) -> q (scalar last)1/1, Unit Delay/1

== system mySAD_project_full_mission/Attitude determination and sensoring/Subsystem1/Switch Case Action Triad Case/TRIAD: Attitude determination algebric Method with 2 sensor ==
  note: 𝑉^(-1) = 𝑉';
      | 𝐴 = 𝑆𝑉^(-1) = 𝑆𝑉'
  note: 𝑣1 = 𝑎;
      | 𝑣2 = (𝑎 ∧ 𝑏)/|𝑎 ∧ 𝑏|;
      | 𝑣3 = 𝑎 ∧ 𝑣2
  note: S1 = 𝑝;
      | 𝑠2 = (𝑝 ∧ 𝑞)/(|𝑝 ∧ 𝑞|);
      | 𝑠3 = 𝑝 ∧ 𝑠2
  Sensor1 (body frame) : Inport
  Sensor2 (body frame) : Inport  Port=2
  Reference1 (Inertial frame) : Inport  Port=3
  Reference2 (Inertial frame) : Inport  Port=4
  Matrix Multiply : Product  Multiplication=Matrix(*)
  Normalize Vector1 : Subsystem
  Normalize Vector2 : Subsystem
  Normalize Vector3 : Subsystem
  Normalize Vector4 : Subsystem
  Subsystem : Subsystem
  Subsystem1 : Subsystem
  Transpose : Math  Operator=transpose
  DCM_B/N  Att Det : Outport
  wires:
  Sensor1 (body frame)/1 -> Normalize Vector2/1(Vector)  "q"
  Sensor2 (body frame)/1 -> Normalize Vector3/1(Vector)  "p"
  Subsystem/1("Matrix S Measurements ") -> Matrix Multiply/1  "Matrix S Measurements (body frame)"
  Normalize Vector2/1(Versor) -> Subsystem/1(versor p (body frame))
  Normalize Vector3/1(Versor) -> Subsystem/2(versor q (body frame))
  Reference2 (Inertial frame)/1 -> Normalize Vector4/1(Vector)  "b"
  Reference1 (Inertial frame)/1 -> Normalize Vector1/1(Vector)  "a"
  Subsystem1/1("Matrix V certain model ") -> Transpose/1  "Matrix V (inertial frame)"
  Normalize Vector4/1(Versor) -> Subsystem1/2(versor b (inertial))
  Matrix Multiply/1 -> DCM_B/N  Att Det/1  "DCM_B/N from attirude determination"
  Transpose/1 -> Matrix Multiply/2
  Normalize Vector1/1(Versor) -> Subsystem1/1(versor a (inertial))

== system mySAD_project_full_mission/Calculation of disturbance torque/Solar pressure on 6 faces/Solar pressure on 6 faces1/Norm of vector ==
  Vector : Inport
  Dot Product : DotProduct  OutDataTypeStr=Inherit: Inherit via internal rule
  Sqrt : Sqrt
  Norm : Outport
  wires:
  Sqrt/1 -> Norm/1
  Vector/1 -> Dot Product/1, Dot Product/2
  Dot Product/1 -> Sqrt/1

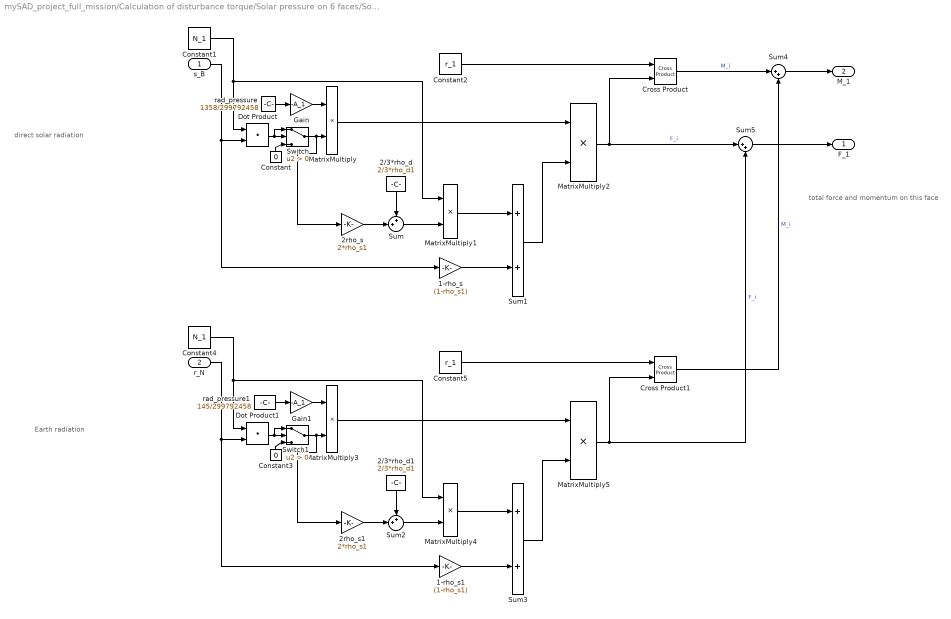
== system mySAD_project_full_mission/Calculation of disturbance torque/Solar pressure on 6 faces/Solar pressure on 6 faces1/solar pressure force and torque 1 ==
  note: total force and
      | momentum on this face
  note: direct solar radiation
  note: Earth radiation
  s_B : Inport
  r_N : Inport  Port=2
  1-rho_s : Gain  Gain=(1-rho_s1)
  1-rho_s1 : Gain  Gain=(1-rho_s1)
  2/3*rho_d : Constant  Value=2/3*rho_d1
  2/3*rho_d1 : Constant  Value=2/3*rho_d1
  2rho_s : Gain  Gain=2*rho_s1
  2rho_s1 : Gain  Gain=2*rho_s1
  Constant : Constant  Value=0
  Constant1 : Constant  Value=N_1
  Constant2 : Constant  Value=r_1
  Constant3 : Constant  Value=0
  Constant4 : Constant  Value=N_1
  Constant5 : Constant  Value=r_1
  Cross Product : matrix_library/Cross Product
  Cross Product1 : matrix_library/Cross Product
  Dot Product : DotProduct  OutDataTypeStr=Inherit: Inherit via internal rule
  Dot Product1 : DotProduct  OutDataTypeStr=Inherit: Inherit via internal rule
  Gain : Gain  Gain=-A_1
  Gain1 : Gain  Gain=-A_1
  MatrixMultiply{,1..5} (6 alike) : Product
  Sum : Sum  Inputs=++|
  Sum1 : Sum
  Sum2 : Sum  Inputs=++|
  Sum3 : Sum
  Sum4 : Sum  Inputs=|++
  Sum5 : Sum  Inputs=|++
  Switch : Switch  Criteria=u2 > Threshold  SaturateOnIntegerOverflow=off  InputSameDT=off
  Switch1 : Switch  Criteria=u2 > Threshold  SaturateOnIntegerOverflow=off  InputSameDT=off
  rad_pressure : Constant  Value=1358/299792458
  rad_pressure1 : Constant  Value=145/299792458
  F_1 : Outport
  M_1 : Outport  Port=2
  wires:
  MatrixMultiply2/1 -> Sum5/1, Cross Product/2  "F_i"
  MatrixMultiply/1 -> MatrixMultiply2/1
  Sum1/1 -> MatrixMultiply2/2
  s_B/1 -> 1-rho_s/1, Dot Product/2
  1-rho_s/1 -> Sum1/2
  rad_pressure/1 -> Gain/1
  MatrixMultiply1/1 -> Sum1/1
  Constant1/1 -> MatrixMultiply1/1, Dot Product/1
  Gain/1 -> MatrixMultiply/1
  Constant2/1 -> Cross Product/1
  Dot Product/1 -> Switch/1, Switch/2
  Constant/1 -> Switch/3
  Switch/1 -> 2rho_s/1, MatrixMultiply/2
  2rho_s/1 -> Sum/2
  2/3*rho_d/1 -> Sum/1
  Sum/1 -> MatrixMultiply1/2
  Sum3/1 -> MatrixMultiply5/2
  r_N/1 -> 1-rho_s1/1, Dot Product1/2
  1-rho_s1/1 -> Sum3/2
  2rho_s1/1 -> Sum2/2
  Switch1/1 -> 2rho_s1/1, MatrixMultiply3/2
  MatrixMultiply4/1 -> Sum3/1
  Constant5/1 -> Cross Product1/1
  MatrixMultiply3/1 -> MatrixMultiply5/1
  rad_pressure1/1 -> Gain1/1
  Constant3/1 -> Switch1/3
  Constant4/1 -> MatrixMultiply4/1, Dot Product1/1
  MatrixMultiply5/1 -> Sum5/2, Cross Product1/2  "F_i"
  Dot Product1/1 -> Switch1/1, Switch1/2
  Cross Product1/1 -> Sum4/2  "M_i"
  Sum2/1 -> MatrixMultiply4/2
  Gain1/1 -> MatrixMultiply3/1
  2/3*rho_d1/1 -> Sum2/1
  Sum4/1 -> M_1/1
  Cross Product/1 -> Sum4/1  "M_i"
  Sum5/1 -> F_1/1

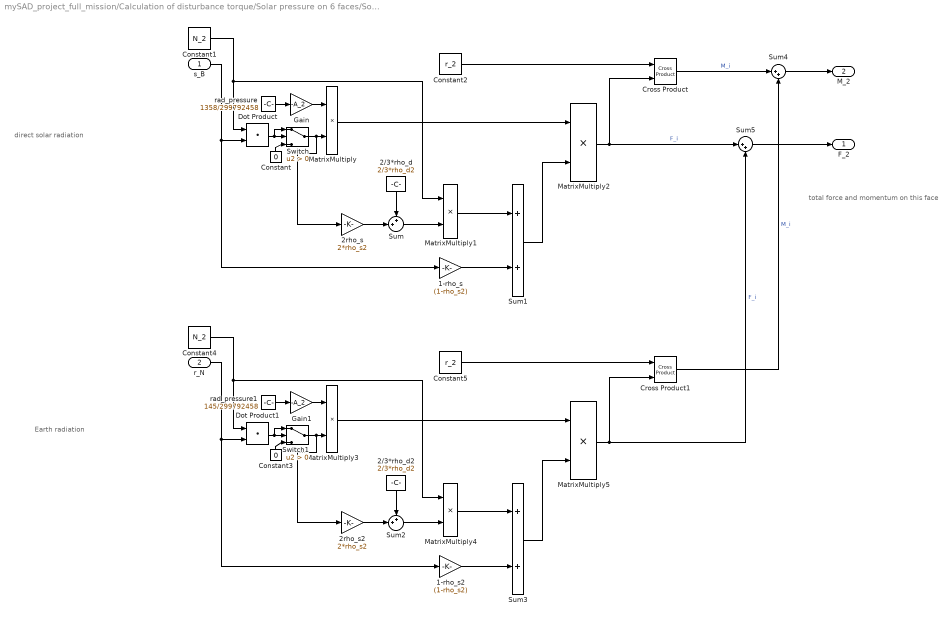
== system mySAD_project_full_mission/Calculation of disturbance torque/Solar pressure on 6 faces/Solar pressure on 6 faces1/solar pressure force and torque 2 ==
  note: total force and
      | momentum on this face
  note: direct solar radiation
  note: Earth radiation
  s_B : Inport
  r_N : Inport  Port=2
  1-rho_s : Gain  Gain=(1-rho_s2)
  1-rho_s2 : Gain  Gain=(1-rho_s2)
  2/3*rho_d : Constant  Value=2/3*rho_d2
  2/3*rho_d2 : Constant  Value=2/3*rho_d2
  2rho_s : Gain  Gain=2*rho_s2
  2rho_s2 : Gain  Gain=2*rho_s2
  Constant : Constant  Value=0
  Constant1 : Constant  Value=N_2
  Constant2 : Constant  Value=r_2
  Constant3 : Constant  Value=0
  Constant4 : Constant  Value=N_2
  Constant5 : Constant  Value=r_2
  Cross Product : matrix_library/Cross Product
  Cross Product1 : matrix_library/Cross Product
  Dot Product : DotProduct  OutDataTypeStr=Inherit: Inherit via internal rule
  Dot Product1 : DotProduct  OutDataTypeStr=Inherit: Inherit via internal rule
  Gain : Gain  Gain=-A_2
  Gain1 : Gain  Gain=-A_2
  MatrixMultiply{,1..5} (6 alike) : Product
  Sum : Sum  Inputs=++|
  Sum1 : Sum
  Sum2 : Sum  Inputs=++|
  Sum3 : Sum
  Sum4 : Sum  Inputs=|++
  Sum5 : Sum  Inputs=|++
  Switch : Switch  Criteria=u2 > Threshold  SaturateOnIntegerOverflow=off  InputSameDT=off
  Switch1 : Switch  Criteria=u2 > Threshold  SaturateOnIntegerOverflow=off  InputSameDT=off
  rad_pressure : Constant  Value=1358/299792458
  rad_pressure1 : Constant  Value=145/299792458
  F_2 : Outport
  M_2 : Outport  Port=2
  wires:
  MatrixMultiply2/1 -> Sum5/1, Cross Product/2  "F_i"
  MatrixMultiply/1 -> MatrixMultiply2/1
  Sum1/1 -> MatrixMultiply2/2
  s_B/1 -> 1-rho_s/1, Dot Product/2
  1-rho_s/1 -> Sum1/2
  rad_pressure/1 -> Gain/1
  MatrixMultiply1/1 -> Sum1/1
  Constant1/1 -> MatrixMultiply1/1, Dot Product/1
  Gain/1 -> MatrixMultiply/1
  Constant2/1 -> Cross Product/1
  Dot Product/1 -> Switch/1, Switch/2
  Constant/1 -> Switch/3
  Switch/1 -> 2rho_s/1, MatrixMultiply/2
  2rho_s/1 -> Sum/2
  2/3*rho_d/1 -> Sum/1
  Sum/1 -> MatrixMultiply1/2
  Sum3/1 -> MatrixMultiply5/2
  r_N/1 -> 1-rho_s2/1, Dot Product1/2
  1-rho_s2/1 -> Sum3/2
  2rho_s2/1 -> Sum2/2
  Switch1/1 -> 2rho_s2/1, MatrixMultiply3/2
  MatrixMultiply4/1 -> Sum3/1
  Constant5/1 -> Cross Product1/1
  MatrixMultiply3/1 -> MatrixMultiply5/1
  rad_pressure1/1 -> Gain1/1
  Constant3/1 -> Switch1/3
  Constant4/1 -> MatrixMultiply4/1, Dot Product1/1
  MatrixMultiply5/1 -> Sum5/2, Cross Product1/2  "F_i"
  Dot Product1/1 -> Switch1/1, Switch1/2
  Cross Product1/1 -> Sum4/2  "M_i"
  Sum2/1 -> MatrixMultiply4/2
  Gain1/1 -> MatrixMultiply3/1
  2/3*rho_d2/1 -> Sum2/1
  Sum4/1 -> M_2/1
  Cross Product/1 -> Sum4/1  "M_i"
  Sum5/1 -> F_2/1

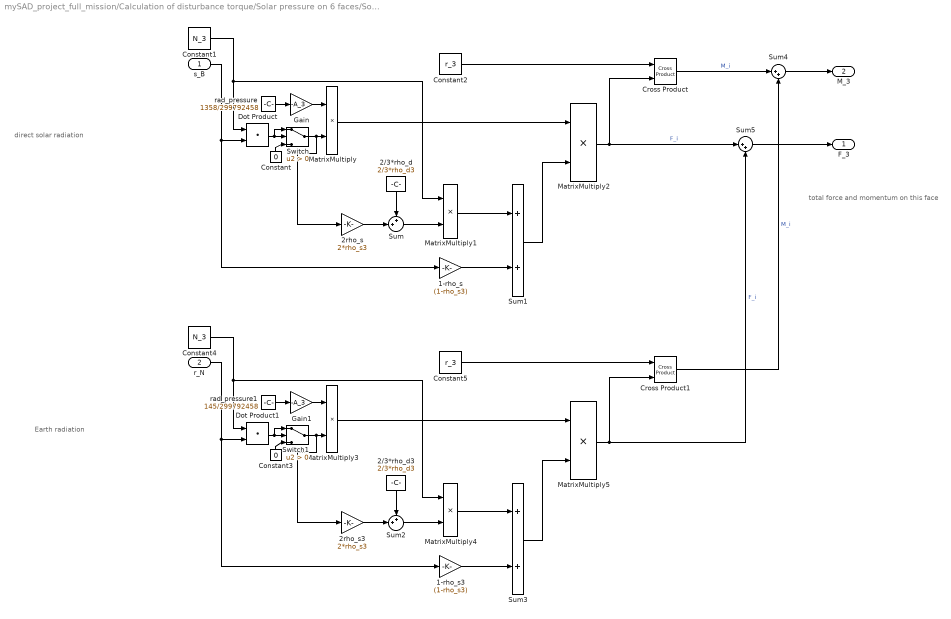
== system mySAD_project_full_mission/Calculation of disturbance torque/Solar pressure on 6 faces/Solar pressure on 6 faces1/solar pressure force and torque 3 ==
  note: total force and
      | momentum on this face
  note: direct solar radiation
  note: Earth radiation
  s_B : Inport
  r_N : Inport  Port=2
  1-rho_s : Gain  Gain=(1-rho_s3)
  1-rho_s3 : Gain  Gain=(1-rho_s3)
  2/3*rho_d : Constant  Value=2/3*rho_d3
  2/3*rho_d3 : Constant  Value=2/3*rho_d3
  2rho_s : Gain  Gain=2*rho_s3
  2rho_s3 : Gain  Gain=2*rho_s3
  Constant : Constant  Value=0
  Constant1 : Constant  Value=N_3
  Constant2 : Constant  Value=r_3
  Constant3 : Constant  Value=0
  Constant4 : Constant  Value=N_3
  Constant5 : Constant  Value=r_3
  Cross Product : matrix_library/Cross Product
  Cross Product1 : matrix_library/Cross Product
  Dot Product : DotProduct  OutDataTypeStr=Inherit: Inherit via internal rule
  Dot Product1 : DotProduct  OutDataTypeStr=Inherit: Inherit via internal rule
  Gain : Gain  Gain=-A_3
  Gain1 : Gain  Gain=-A_3
  MatrixMultiply{,1..5} (6 alike) : Product
  Sum : Sum  Inputs=++|
  Sum1 : Sum
  Sum2 : Sum  Inputs=++|
  Sum3 : Sum
  Sum4 : Sum  Inputs=|++
  Sum5 : Sum  Inputs=|++
  Switch : Switch  Criteria=u2 > Threshold  SaturateOnIntegerOverflow=off  InputSameDT=off
  Switch1 : Switch  Criteria=u2 > Threshold  SaturateOnIntegerOverflow=off  InputSameDT=off
  rad_pressure : Constant  Value=1358/299792458
  rad_pressure1 : Constant  Value=145/299792458
  F_3 : Outport
  M_3 : Outport  Port=2
  wires:
  MatrixMultiply2/1 -> Sum5/1, Cross Product/2  "F_i"
  MatrixMultiply/1 -> MatrixMultiply2/1
  Sum1/1 -> MatrixMultiply2/2
  s_B/1 -> 1-rho_s/1, Dot Product/2
  1-rho_s/1 -> Sum1/2
  rad_pressure/1 -> Gain/1
  MatrixMultiply1/1 -> Sum1/1
  Constant1/1 -> MatrixMultiply1/1, Dot Product/1
  Gain/1 -> MatrixMultiply/1
  Constant2/1 -> Cross Product/1
  Dot Product/1 -> Switch/1, Switch/2
  Constant/1 -> Switch/3
  Switch/1 -> 2rho_s/1, MatrixMultiply/2
  2rho_s/1 -> Sum/2
  2/3*rho_d/1 -> Sum/1
  Sum/1 -> MatrixMultiply1/2
  Sum3/1 -> MatrixMultiply5/2
  r_N/1 -> 1-rho_s3/1, Dot Product1/2
  1-rho_s3/1 -> Sum3/2
  2rho_s3/1 -> Sum2/2
  Switch1/1 -> 2rho_s3/1, MatrixMultiply3/2
  MatrixMultiply4/1 -> Sum3/1
  Constant5/1 -> Cross Product1/1
  MatrixMultiply3/1 -> MatrixMultiply5/1
  rad_pressure1/1 -> Gain1/1
  Constant3/1 -> Switch1/3
  Constant4/1 -> MatrixMultiply4/1, Dot Product1/1
  MatrixMultiply5/1 -> Sum5/2, Cross Product1/2  "F_i"
  Dot Product1/1 -> Switch1/1, Switch1/2
  Cross Product1/1 -> Sum4/2  "M_i"
  Sum2/1 -> MatrixMultiply4/2
  Gain1/1 -> MatrixMultiply3/1
  2/3*rho_d3/1 -> Sum2/1
  Sum4/1 -> M_3/1
  Cross Product/1 -> Sum4/1  "M_i"
  Sum5/1 -> F_3/1
